simulink model "PreCondition"  (R2018b)
settings: Solver=FixedStepDiscrete  StartTime=0.0  StopTime=10.0  FixedStep=0.01  RelTol=1e-3
undefined symbols (not defined in the file or in its folder): EnergyMgLdShdRq1, HMI_2L_StMd10_Config_Val, HMI_2L_StMd11_Config_Val, HMI_2L_StMd12_Config_Val, HMI_2L_StMd13_Config_Val, HMI_2L_StMd14_Config_Val, HMI_2L_StMd15_Config_Val, HMI_2L_StMd16_Config_Val, HMI_2L_StMd17_Config_Val, HMI_2L_StMd18_Config_Val, HMI_2L_StMd19_Config_Val, HMI_2L_StMd1_Config_Val, HMI_2L_StMd20_Config_Val, HMI_2L_StMd21_Config_Val, HMI_2L_StMd22_Config_Val, HMI_2L_StMd23_Config_Val, HMI_2L_StMd24_Config_Val, HMI_2L_StMd25_Config_Val, HMI_2L_StMd26_Config_Val, HMI_2L_StMd27_Config_Val, HMI_2L_StMd28_Config_Val, HMI_2L_StMd29_Config_Val, HMI_2L_StMd2_Config_Val, HMI_2L_StMd30_Config_Val, HMI_2L_StMd31_Config_Val, HMI_2L_StMd32_Config_Val, HMI_2L_StMd3_Config_Val, HMI_2L_StMd4_Config_Val, HMI_2L_StMd5_Config_Val, HMI_2L_StMd6_Config_Val, HMI_2L_StMd7_Config_Val, HMI_2L_StMd8_Config_Val, HMI_2L_StMd9_Config_Val, HMI_2R_StMd10_Config_Val, HMI_2R_StMd11_Config_Val, HMI_2R_StMd12_Config_Val, HMI_2R_StMd13_Config_Val, HMI_2R_StMd14_Config_Val, HMI_2R_StMd15_Config_Val, HMI_2R_StMd16_Config_Val, HMI_2R_StMd17_Config_Val, HMI_2R_StMd18_Config_Val, HMI_2R_StMd19_Config_Val, HMI_2R_StMd1_Config_Val, HMI_2R_StMd20_Config_Val, HMI_2R_StMd21_Config_Val, HMI_2R_StMd22_Config_Val, HMI_2R_StMd23_Config_Val, HMI_2R_StMd24_Config_Val, HMI_2R_StMd25_Config_Val, HMI_2R_StMd26_Config_Val, HMI_2R_StMd27_Config_Val, HMI_2R_StMd28_Config_Val, HMI_2R_StMd29_Config_Val, HMI_2R_StMd2_Config_Val, HMI_2R_StMd30_Config_Val, HMI_2R_StMd31_Config_Val, HMI_2R_StMd32_Config_Val, HMI_2R_StMd3_Config_Val, HMI_2R_StMd4_Config_Val ... (+94)
(part 2 of 6)

== system PreCondition/PreCondition_Init ==
  Event Listener : EventListener  EventName=reset
